simulink model "realtimeModel"  (R2024b)
settings: Solver=ode5  StartTime=0.0  StopTime=sIn.t_sim  FixedStep=0.001  RelTol=1e-3
values from neighbouring files (symbols this model uses):
  PID = computePIDGains(8, 0.15, 0.1, plant.Ps, "PID")    [lab0_startup.m]
undefined symbols (not defined in the file or in its folder): degs2rpm, filt, gbox, National_Instruments, PCIe, rpm2degs, sens, sIn
libraries: simulink x3, sldrtlib x3, simulink_extras x1
settings Model: SimulationMode=external  ExtModeTrigDuration=20001  Creator=surinihal  LastModifiedBy=surinihal
settings HardwareCC: ProdBitPerLong=64  ProdHWDeviceType=Intel->x86-64 (Linux 64)
settings RTWCC: Description=Simulink Desktop Real-Time  SystemTargetFile=sldrt.tlc  TemplateMakefile=sldrt.tmf  RTWCompilerOptimization=on
settings CodeAppCC: MaxIdLength=95
settings SimulinkDesktopRealTimeCC: TargetLibSuffix=_sldrt.a  TargetPreCompLibLocation=C:\Program Files\MATLAB\R2024b\toolbox\sldrt\lib\win64  ParMdlRefBuildCompliant=on

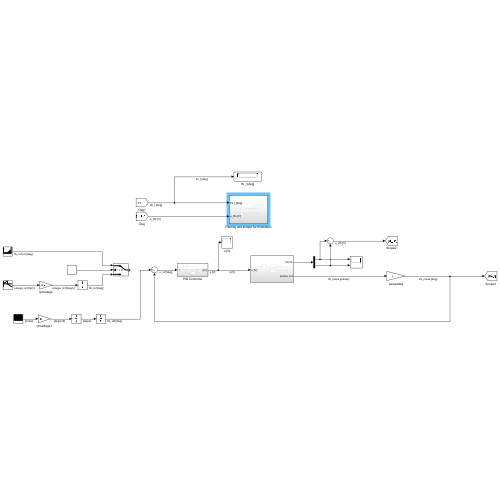
[thumbnail: Simulink's stored preview of the top-level diagram]
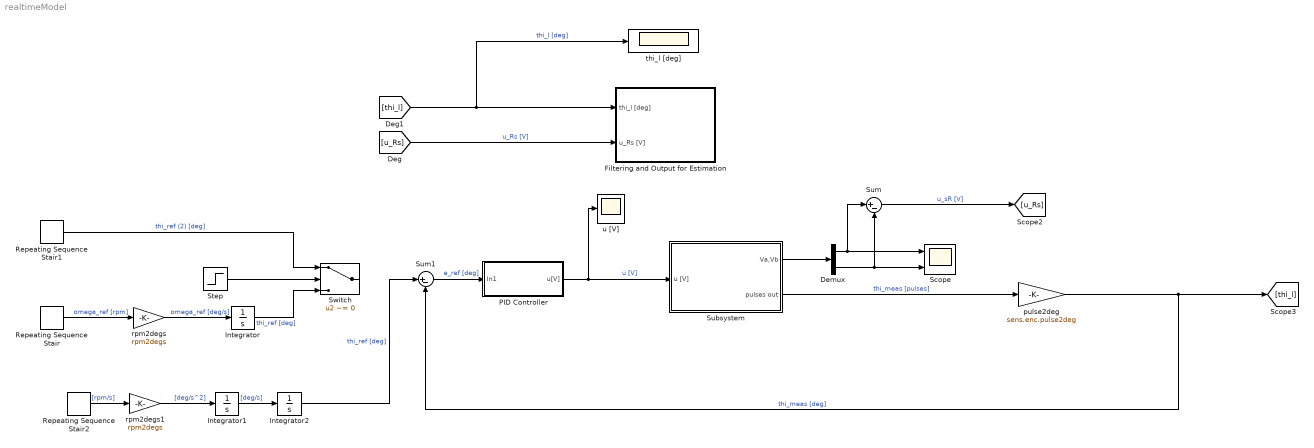
== system realtimeModel ==
  Demux : Demux  Outputs=2
  Filtering and Output for Estimation : Subsystem
  Integrator : Integrator
  Integrator1 : Integrator
  Integrator2 : Integrator
  PID Controller : Subsystem
  Repeating Sequence Stair : simulink/Sources/Repeating Sequence Stair  OutValues=sIn.omega_l  tsamp=sIn.step_time  OutMin=[]  OutMax=[]  OutDataTypeStr=double  OutputDataTypeScalingMode=double  OutDataType=fixdt(0,8)  ConRadixGroup=Best Precision: Vector-wise  OutScaling=2^-12
  Repeating Sequence Stair1 : simulink/Sources/Repeating Sequence Stair  OutValues=sIn.resp  tsamp=sIn.length_steps  OutMin=[]  OutMax=[]  OutDataTypeStr=double  OutputDataTypeScalingMode=double  OutDataType=fixdt(0,8)  ConRadixGroup=Best Precision: Vector-wise  OutScaling=2^-12
  Repeating Sequence Stair2 : simulink/Sources/Repeating Sequence Stair  OutValues=sIn.A  tsamp=sIn.acc_step_time  OutMin=[]  OutMax=[]  OutDataTypeStr=double  OutputDataTypeScalingMode=double  OutDataType=fixdt(0,8)  ConRadixGroup=Best Precision: Vector-wise  OutScaling=2^-12
  Scope : Scope  NumInputPorts=2
  Step : Step  Time=0  After=sIn.pid  SampleTime=0
  Subsystem : Subsystem
  Sum : Sum  Inputs=|+-
  Sum1 : Sum  Inputs=|+-
  Switch : Switch  Criteria=u2 ~= 0  SaturateOnIntegerOverflow=off  InputSameDT=off
  pulse2deg : Gain  Gain=sens.enc.pulse2deg
  rpm2degs : Gain  Gain=rpm2degs
  rpm2degs1 : Gain  Gain=rpm2degs
  thi_l [deg] : Scope
  u [V] : Scope
  wires:
  Demux/1 -> Sum/1, Scope/1
  Demux/2 -> Scope/2, Sum/2
  Sum/1 -> [u_Rs]  "u_sR [V]"
  PID Controller/1(u[V]) -> Subsystem/1(u [V]), u [V]/1  "u [V]"
  Subsystem/1(Va,Vb) -> Demux/1
  Subsystem/2(pulses out) -> pulse2deg/1  "thi_meas [pulses]"
  pulse2deg/1 -> [thi_l], Sum1/2  "thi_meas [deg]"
  Repeating Sequence Stair1/1 -> Switch/1  "thi_ref (2) [deg]"
  Integrator/1 -> Switch/3  "thi_ref [deg]"
  Step/1 -> Switch/2
  [thi_l] -> thi_l [deg]/1, Filtering and Output for Estimation/1(thi_l [deg])  "thi_l [deg]"
  rpm2degs/1 -> Integrator/1  "omega_ref [deg/s]"
  Repeating Sequence Stair/1 -> rpm2degs/1  "omega_ref [rpm]"
  [u_Rs] -> Filtering and Output for Estimation/2(u_Rs [V])  "u_Rs [V]"
  Sum1/1 -> PID Controller/1(In1)  "e_ref [deg]"
  Repeating Sequence Stair2/1 -> rpm2degs1/1  "[rpm/s]"
  rpm2degs1/1 -> Integrator1/1  "[deg/s^2]"
  Integrator1/1 -> Integrator2/1  "[deg/s]"
  Integrator2/1 -> Sum1/1  "thi_ref [deg]"

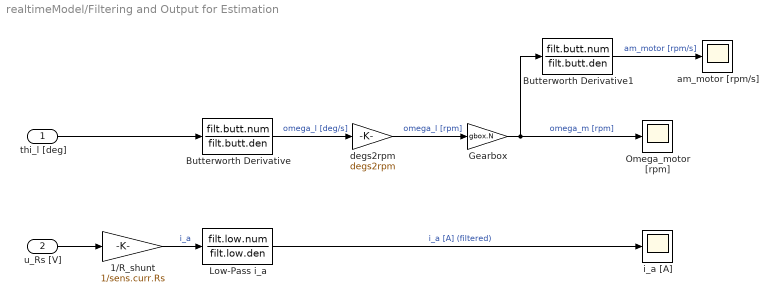
== system realtimeModel/Filtering and Output for Estimation ==
  thi_l [deg] : Inport
  u_Rs [V] : Inport  Port=2
  1/R_shunt : Gain  Gain=1/sens.curr.Rs
  Butterworth Derivative : TransferFcn  Numerator=filt.butt.num  Denominator=filt.butt.den
  Butterworth Derivative1 : TransferFcn  Numerator=filt.butt.num  Denominator=filt.butt.den
  Gearbox : Gain  Gain=gbox.N
  Low-Pass i_a : TransferFcn  Numerator=filt.low.num  Denominator=filt.low.den
  Omega_motor [rpm] : Scope
  am_motor [rpm/s] : Scope
  degs2rpm : Gain  Gain=degs2rpm
  i_a [A] : Scope
  wires:
  1/R_shunt/1 -> Low-Pass i_a/1  "i_a"
  Gearbox/1 -> Butterworth Derivative1/1, Omega_motor [rpm]/1  "omega_m [rpm]"
  Butterworth Derivative/1 -> degs2rpm/1  "omega_l [deg/s]"
  degs2rpm/1 -> Gearbox/1  "omega_l [rpm]"
  u_Rs [V]/1 -> 1/R_shunt/1
  Low-Pass i_a/1 -> i_a [A]/1  "i_a [A] (filtered)"
  thi_l [deg]/1 -> Butterworth Derivative/1
  Butterworth Derivative1/1 -> am_motor [rpm/s]/1  "am_motor [rpm/s]"

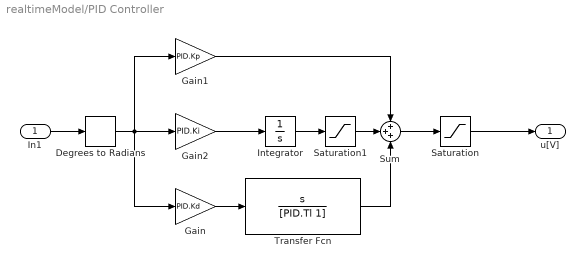
== system realtimeModel/PID Controller ==
  In1 : Inport
  Degrees to Radians : simulink_extras/Transformations/Degrees to Radians
  Gain : Gain  Gain=PID.Kd
  Gain1 : Gain  Gain=PID.Kp
  Gain2 : Gain  Gain=PID.Ki
  Integrator : Integrator
  Saturation : Saturate  UpperLimit=10  LowerLimit=-10
  Saturation1 : Saturate  UpperLimit=PID.i_saturation  LowerLimit=-PID.i_saturation
  Sum : Sum  Inputs=+++
  Transfer Fcn : TransferFcn  Numerator=[1 0]  Denominator=[PID.Tl 1]
  u[V] : Outport
  wires:
  In1/1 -> Degrees to Radians/1
  Sum/1 -> Saturation/1
  Saturation/1 -> u[V]/1
  Degrees to Radians/1 -> Gain/1, Gain1/1, Gain2/1
  Gain/1 -> Transfer Fcn/1
  Gain2/1 -> Integrator/1
  Transfer Fcn/1 -> Sum/3
  Integrator/1 -> Saturation1/1
  Gain1/1 -> Sum/1
  Saturation1/1 -> Sum/2

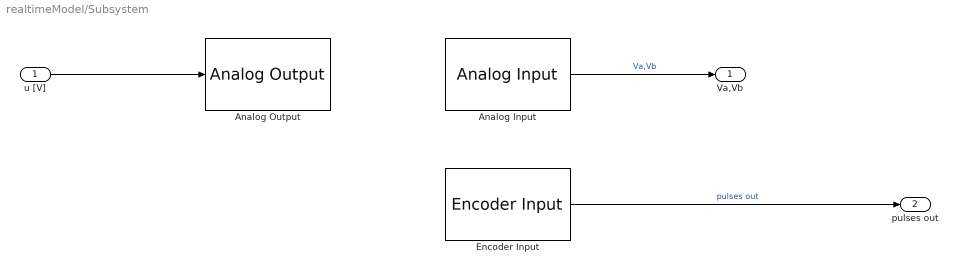
== system realtimeModel/Subsystem ==
  u [V] : Inport
  Analog Input : sldrtlib/Analog Input  SampleTime=-1  MaxMissedTicks=10  ShowMissedTicks=off  YieldWhenWaiting=off  DrvName=National_Instruments/PCIe-6321  DrvAddress=4294967295  DrvOptions=[0 0 0 2 0 0 0]  Channels=[1,2]  RangeMode=1  VoltRange=1  DataType=1
      settings: AttributesFormatString=National Instruments\nPCIe-6321 [auto]
  Analog Output : sldrtlib/Analog Output  SampleTime=-1  MaxMissedTicks=10  ShowMissedTicks=off  YieldWhenWaiting=off  DrvName=National_Instruments/PCIe-6321  DrvAddress=4294967295  DrvOptions=[0 0 0 2 0 0 0]  Channels=1  RangeMode=1  VoltRange=1  InitialValue=0  FinalValue=0
      settings: AttributesFormatString=National Instruments\nPCIe-6321 [auto]
  Encoder Input : sldrtlib/Encoder Input  SampleTime=-1  MaxMissedTicks=10  ShowMissedTicks=off  YieldWhenWaiting=off  DrvName=National_Instruments/PCIe-6321  DrvAddress=4294967295  DrvOptions=[0 0 0 2 0 0 0]  Channels=1  QuadMode=3  IndexPulse=1  InputFilter=Inf  DataType=1
      settings: AttributesFormatString=National Instruments\nPCIe-6321 [auto]
  Va,Vb : Outport
  pulses out : Outport  Port=2
  wires:
  Encoder Input/1 -> pulses out/1  "pulses out"
  Analog Input/1 -> Va,Vb/1  "Va,Vb"
  u [V]/1 -> Analog Output/1
